simulink model "Skills_Team_15801E_2024"  (R2023a)
settings: Solver=FixedStepAuto  StartTime=0.0  StopTime=inf  RelTol=1e-3
libraries: vexv5lib x45, vexcommonlib x3, slpidlib x2
settings Model: Creator=ctwildnauer24  LastModifiedBy=kevans
settings OptimizationCC: EnhancedBackFolding=on  PassReuseOutputArgsAs=Individual arguments  ZeroExternalMemoryAtStartup=off  ZeroInternalMemoryAtStartup=off  MaxStackSize=64  OptimizeBlockOrder=speed  DifferentSizesBufferReuse=on  OptimizationCustomize=off  EfficientTunableParamExpr=on
settings DebuggingCC: ParameterTunabilityLossMsg=error
settings HardwareCC: ProdBitPerPointer=32  ProdBitPerSizeT=32  ProdBitPerPtrDiffT=32  ProdLargestAtomicInteger=Long  ProdLargestAtomicFloat=Double  ProdWordSize=32  ProdHWDeviceType=ARM Compatible->ARM Cortex  UseEmbeddedCoderFeatures=off
settings SFSimCC: MATLABDynamicMemAlloc=off
settings RTWCC: Description=Embedded Coder  SystemTargetFile=ert.tlc  HardwareBoard=VEX V5 Robot Brain  TLCOptions="-aInlineSetEventsForThisBaseRateFcn=TLC_FALSE -aSuppressMultiTaskScheduler=TLC_FALSE  -aRateBasedStepFcn=0"  TemplateMakefile=ert_default_tmf  Toolchain=GNU Tools for ARM Embedded Processors
settings CodeAppCC: ForceParamTrailComments=on  IgnoreCustomStorageClasses=off  OperatorAnnotations=on  SimulinkDataObjDesc=on  SFDataObjDesc=on  InsertBlockDesc=on
settings ERTTargetCC: SupportNonInlinedSFcns=on  ExtModeTransport=3  ExtModeStaticAlloc=on  ExtModeStaticAllocSize=2048  ExtModeMexFile=ext_xcp  ExtModeIntrfLevel=Level2 - Open

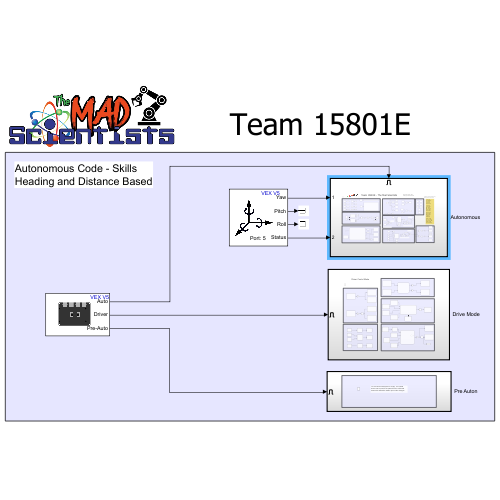
[thumbnail: Simulink's stored preview of the top-level diagram]
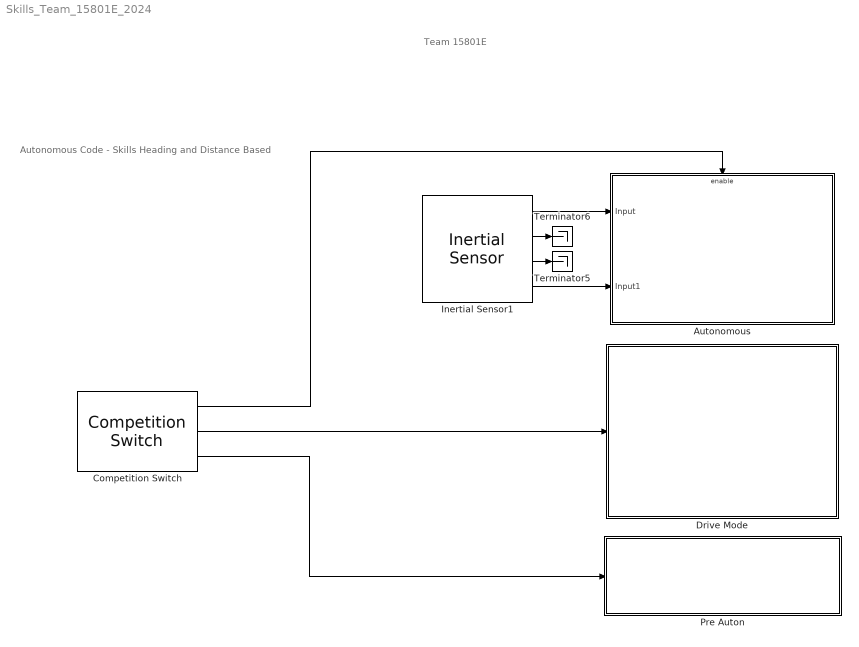
== system Skills_Team_15801E_2024 ==
  note: Team 15801E
  note: Autonomous Code - Skills
      | Heading and Distance Based
  "Autonomous " : Subsystem  TreatAsAtomicUnit=on
  Competition Switch : vexv5lib/Gamepad/Competition Switch  SampleTime=0.02
  "Drive Mode " : Subsystem  TreatAsAtomicUnit=on
  Inertial Sensor1 : vexv5lib/Sensors/Inertial Sensor  Port=5  ypr=on  Quat=off  AngVel=off  Accel=off  CalibStatus=on  YawResetOption=No reset  YawWrapAround=No wrap around  SampleTime=.01
  Pre Auton : Subsystem  TreatAsAtomicUnit=on
  Terminator5 : Terminator
  Terminator6 : Terminator
  wires:
  Competition Switch/2 -> "Drive Mode "/Enable
  Competition Switch/3 -> Pre Auton/Enable
  Competition Switch/1 -> "Autonomous "/Enable
  Inertial Sensor1/3 -> Terminator5/1
  Inertial Sensor1/2 -> Terminator6/1
  Inertial Sensor1/4 -> "Autonomous "/2(Input1)
  Inertial Sensor1/1 -> "Autonomous "/1(Input)

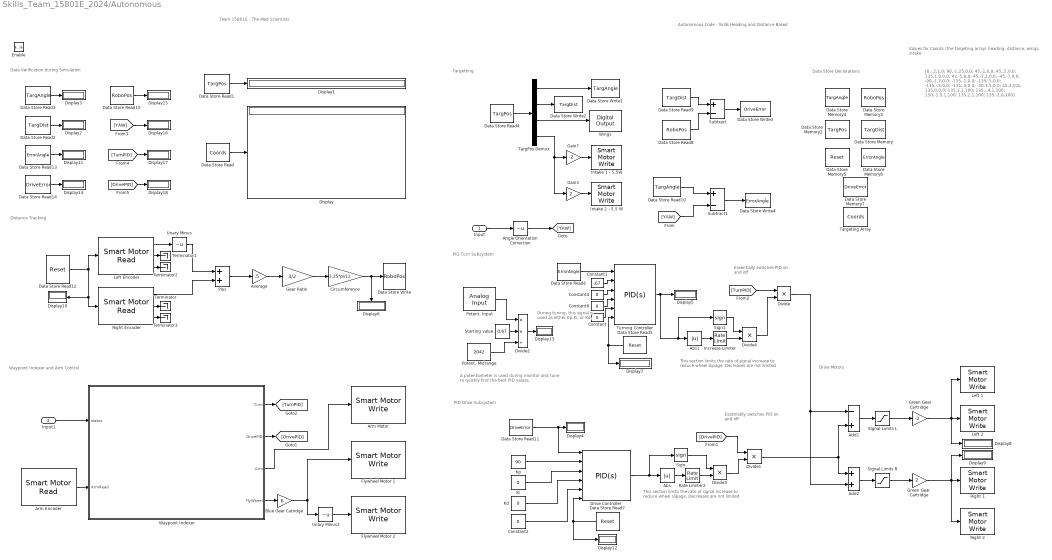
== system Skills_Team_15801E_2024/Autonomous  ==
  note: A potentiometer is used during monitor and tune to quickly find the best PID values.
  note: Data Verification during Simulation
  note: Data Store Declarations
  note: Drive Motors
  note: Waypoint Indexer and Arm Control
  note: Distance Tracking
  note: Team 15801E - The Mad Scientists
  note: PID Turn Subsystem
  note: Autonomous Code - Skills
      | Heading and Distance Based
  note: [0,-.2,1,0;
      | 90,-1.25,0,0;
      | 45,-1,0,0;
      | 45,.5,0,0;
      | 135,1.9,0,0;
      | 42,-5,0,0;
      | 45,-3.2,0,0;
      | -45,-7,0,0;
      | -90,-1.7,0,0;
      | -135,-1,0,0;
      | -135,.5,0,0;
      | -135,-.5,0,0;
      | -135,.5,0,0;
      | -30,3.5,0,0;
      | 45,2,0,0;
      | 135,0,0,0;
      | 135,3,1,100;
      | 135,-.4,1,100;
      | 150,-1.5,1,100;
      | 135,2,1,100;
      | 135,-2,0,100]
  note: Targetting
  note: PID Drive Subsystem
  note: Values for Coords (the targeting array)
      | heading, distance, wings, intake
  note: During tuning, this signal is used as either Kp,Ki, or Kd.
  note: This section limits the rate of signal increase to reduce wheel slipage. Decreases are not limited
  note: Essentially switches PID on and off
  note: This section limits the rate of signal increase to reduce wheel slipage. Decreases are not limited
  note: Essentially switches PID on and off
  Input : Inport
  Input1 : Inport  Port=2
  Enable : EnablePort
  - Green Gear Cartridge : Gain  Gain=-2
  Abs : Abs  SaturateOnIntegerOverflow=off
  Abs1 : Abs  SaturateOnIntegerOverflow=off
  Add1 : Sum  Inputs=-+
  Add2 : Sum
  Angle Orientation Correction : UnaryMinus
  Arm Encoder : vexv5lib/Sensors/Smart Motor Read  motorPort=17  EncoderUnit=Degrees  resetOption=No reset  additionalOutput=off  SampleTime=0.2
  Arm Motor : vexv5lib/Actuators/Smart Motor Write  motorPort=17  scaleFactor=36:1  MotorBrakeMode=Coast  OperationMode=Velocity Control
  Average : Gain  Gain=.5
  Blue Gear Catridge : Gain  Gain=6
  Circumference : Gain  Gain=3.25*pi/12
  Constant{,2,4,6} (4 alike) : Constant  Value=0
  Constant1 : Constant  Value=.67
  Data Store Memory : DataStoreMemory  DataStoreName=TargDist  WriteAfterWriteMsg=warning  ShowAdditionalParam=off  OutDataTypeStr=double
  Data Store Memory2 : DataStoreMemory  DataStoreName=TargPos  WriteAfterWriteMsg=warning  InitialValue=[0,0,0,0]  ShowAdditionalParam=off  OutDataTypeStr=double
  Data Store Memory3 : DataStoreMemory  DataStoreName=RoboPos  WriteAfterWriteMsg=warning  InitialValue=[0]  ShowAdditionalParam=off  OutDataTypeStr=double
  Data Store Memory4 : DataStoreMemory  DataStoreName=TargAngle  WriteAfterWriteMsg=warning  ShowAdditionalParam=off
  Data Store Memory5 : DataStoreMemory  DataStoreName=Reset  WriteAfterWriteMsg=warning  ShowAdditionalParam=off  OutDataTypeStr=double
  Data Store Memory6 : DataStoreMemory  DataStoreName=ErrorAngle  WriteAfterWriteMsg=warning  ShowAdditionalParam=off  OutDataTypeStr=double
  Data Store Memory7 : DataStoreMemory  DataStoreName=DriveError  WriteAfterWriteMsg=warning  ShowAdditionalParam=off  OutDataTypeStr=double
  Data Store Read : DataStoreRead  DataStoreName=Coords  IndexOptions=Index vector (dialog)  Indices=1  OutputSizes=1
  Data Store Read1 : DataStoreRead  DataStoreName=TargPos  IndexOptions=Index vector (dialog)  Indices=1  OutputSizes=1
  Data Store Read10 : DataStoreRead  DataStoreName=TargAngle  IndexOptions=Index vector (dialog)  Indices=1  OutputSizes=1
  Data Store Read11 : DataStoreRead  DataStoreName=DriveError  IndexOptions=Index vector (dialog)  Indices=1  OutputSizes=1
  Data Store Read12 : DataStoreRead  DataStoreName=Reset  IndexOptions=Index vector (dialog)  Indices=1  OutputSizes=1
  Data Store Read13 : DataStoreRead  DataStoreName=ErrorAngle  IndexOptions=Index vector (dialog)  Indices=1  OutputSizes=1
  Data Store Read14 : DataStoreRead  DataStoreName=DriveError  IndexOptions=Index vector (dialog)  Indices=1  OutputSizes=1
  Data Store Read15 : DataStoreRead  DataStoreName=RoboPos  IndexOptions=Index vector (dialog)  Indices=1  OutputSizes=1
  Data Store Read2 : DataStoreRead  DataStoreName=TargDist  IndexOptions=Index vector (dialog)  Indices=1  OutputSizes=1
  Data Store Read3 : DataStoreRead  DataStoreName=TargAngle  IndexOptions=Index vector (dialog)  Indices=1  OutputSizes=1
  Data Store Read4 : DataStoreRead  DataStoreName=TargPos  IndexOptions=Index vector (dialog)  Indices=1  OutputSizes=1
  Data Store Read5 : DataStoreRead  DataStoreName=Reset  IndexOptions=Index vector (dialog)  Indices=1  OutputSizes=1
  Data Store Read6 : DataStoreRead  DataStoreName=ErrorAngle  IndexOptions=Index vector (dialog)  Indices=1  OutputSizes=1
  Data Store Read7 : DataStoreRead  DataStoreName=Reset  IndexOptions=Index vector (dialog)  Indices=1  OutputSizes=1
  Data Store Read8 : DataStoreRead  DataStoreName=RoboPos  IndexOptions=Index vector (dialog)  Indices=1  OutputSizes=1
  Data Store Read9 : DataStoreRead  DataStoreName=TargDist  IndexOptions=Index vector (dialog)  Indices=1  OutputSizes=1
  Data Store Write : DataStoreWrite  DataStoreName=RoboPos  IndexOptions=Index vector (dialog)  Indices=1  OutputSizes=1
  Data Store Write1 : DataStoreWrite  DataStoreName=TargAngle  IndexOptions=Index vector (dialog)  Indices=1  OutputSizes=1
  Data Store Write2 : DataStoreWrite  DataStoreName=TargDist  IndexOptions=Index vector (dialog)  Indices=1  OutputSizes=1
  Data Store Write3 : DataStoreWrite  DataStoreName=DriveError  IndexOptions=Index vector (dialog)  Indices=1  OutputSizes=1
  Data Store Write4 : DataStoreWrite  DataStoreName=ErrorAngle  IndexOptions=Index vector (dialog)  Indices=1  OutputSizes=1
  Display{,1..18} (19 alike) : Display
  Divide{,1,3..4} (4 alike) : Product  Inputs=**
  Divide2 : Product  Inputs=**/
  Drive Controller : slpidlib/PID Controller  Controller=PID  Form=Parallel  TimeDomain=Continuous-time  UseExternalTs=off  SampleTime=-1  IntegratorMethod=Forward Euler  FilterMethod=Forward Euler  ControllerParametersSource=external  P=40  I=0  UseKiTs=off  D=0  N=100  UseFilter=on  TunerSelectOption=Transfer Function Based (PID Tuner App)  InitialConditionSource=internal  InitialConditionForIntegrator=0  InitialConditionForFilter=0  DifferentiatorICPrevScaledInput=0  ExternalReset=either  TrackingMode=off  Kt=1  LimitOutput=on  SatLimitsSource=internal  UpperSaturationLimit=100  LowerSaturationLimit=-100  LinearizeAsGain=on  AntiWindupMode=none  Kb=1  LimitIntegrator=off  UpperIntegratorSaturationLimit=inf  LowerIntegratorSaturationLimit=-inf  POutMin=[]  POutMax=[]  IOutMin=[]  IOutMax=[]  DOutMin=[]  DOutMax=[]  NOutMin=[]  NOutMax=[]  SumOutMin=[]  SumOutMax=[]  SaturationOutMin=[]  SaturationOutMax=[]  PParamMin=[]  PParamMax=[]  IParamMin=[]  IParamMax=[]  DParamMin=[]  DParamMax=[]  NParamMin=[]  NParamMax=[]  KbParamMin=[]  KbParamMax=[]  KtParamMin=[]  KtParamMax=[]  KbOutMin=[]  KbOutMax=[]  KtOutMin=[]  KtOutMax=[]  IntegratorOutMin=[]  IntegratorOutMax=[]  FilterOutMin=[]  FilterOutMax=[]  SumI1OutMin=[]  SumI1OutMax=[]  SumI2OutMin=[]  SumI2OutMax=[]  SumI3OutMin=[]  SumI3OutMax=[]  SumI4OutMin=[]  SumI4OutMax=[]  SumDOutMin=[]  SumDOutMax=[]  DifferentiatorOutMin=[]  DifferentiatorOutMax=[]  FilterDiffOutCoefMin=[]  FilterDiffOutCoefMax=[]  ReciprocalOutMin=[]  ReciprocalOutMax=[]  SumDenOutMin=[]  SumDenOutMax=[]  SumNumOutMin=[]  SumNumOutMax=[]  DivideOutMin=[]  DivideOutMax=[]  UdiffTsProdOutMin=[]  UdiffTsProdOutMax=[]  NTsProdOutMin=[]  NTsProdOutMax=[]  UintegralTsProdOutMin=[]  UintegralTsProdOutMax=[]  UngainTsProdOutMin=[]  UngainTsProdOutMax=[]  ClampingZeroOutDataTypeStr=Inherit: Inherit via back propagation  ClampingZeroOutMin=[]  ClampingZeroOutMax=[]  FilterDenConstantOutDataTypeStr=Inherit: Inherit via back propagation  FilterDenConstantOutMin=[]  FilterDenConstantOutMax=[]  PCopyOutDataTypeStr=Inherit: Inherit via back propagation  PCopyOutMin=[]  PCopyOutMax=[]  NCopyOutDataTypeStr=Inherit: Inherit via back propagation  NCopyOutMin=[]  NCopyOutMax=[]  IntegratorContinuousStateAttributes=''  IntegratorStateMustResolveToSignalObject=off  IntegratorRTWStateStorageClass=Auto  FilterContinuousStateAttributes=''  FilterStateMustResolveToSignalObject=off  FilterRTWStateStorageClass=Auto  ParallelPVariant=ExternalParameters  IdealPVariant=Disabled  IVariant=ExternalParameters  DVariant=ExternalParameters  IntegratorVariant=Continuous  SatVariant=Enabled  AWVariant=Passthrough  PCopyVariant=Disabled  TRVariant=Disabled  FdbkBlocksVariant=Forward  IdealPFdbkVariant=Disabled  SatFdbkVariant=Disabled  DerivativeFilterVariant=ContFilter  NVariant=ExternalParameters  NCopyVariant=Disabled  FilterICVariant=InternalICsFilter  IntegratorICVariant=InternalICs  ExternalResetVariant=ExternalReset  TRSumVariant=Passthrough  SumFdbkVariant=Disabled  SumVariant=Sum_PID  TsampFilterVariant=InternalTs  TsampNgainVariant=Passthrough  TsampIntegralVariant=Disabled_SignalSpec  ExternalSaturationOutDataTypeStr=Inherit: Same as second input
  Flywheel Motor 1 : vexv5lib/Actuators/Smart Motor Write  motorPort=9  scaleFactor=6:1  MotorBrakeMode=Coast  OperationMode=Velocity Control
  Flywheel Motor 2 : vexv5lib/Actuators/Smart Motor Write  motorPort=20  scaleFactor=6:1  MotorBrakeMode=Coast  OperationMode=Velocity Control
  Gain3 : Gain  Gain=2
  Gain7 : Gain  Gain=-2
  Gear Ratio : Gain  Gain=3/2
  Green Gear Cartridge : Gain  Gain=2
  Increase Limiter : RateLimiter  RisingSlewLimit=80  FallingSlewLimit=-1000000  SampleTimeMode=inherited
  Intake 1 - 5.5W : vexv5lib/Actuators/Smart Motor Write  motorPort=11  scaleFactor=18:1  MotorBrakeMode=Coast  OperationMode=Velocity Control
  Intake 2 - 5.5 W : vexv5lib/Actuators/Smart Motor Write  motorPort=3  scaleFactor=18:1  MotorBrakeMode=Coast  OperationMode=Velocity Control
  Kd : Constant  Value=0
  Ki : Constant  Value=0
  Kp : Constant  Value=90
  Left 1 : vexv5lib/Actuators/Smart Motor Write  motorPort=4  scaleFactor=18:1  MotorBrakeMode=Brake  OperationMode=Velocity Control
  Left 2 : vexv5lib/Actuators/Smart Motor Write  motorPort=1  scaleFactor=18:1  MotorBrakeMode=Brake  OperationMode=Velocity Control
  Left Encoder : vexv5lib/Sensors/Smart Motor Read  motorPort=1  EncoderUnit=Rotations  resetOption=Reset by external signal  additionalOutput=on  SampleTime=.01
  Plus : Sum
  Potent. Input : vexv5lib/Sensors/Analog Input  smartPort3wire=None  port=D  SampleTime=0.2
  Potent. Midrange : Constant  Value=2042
  Rate Limiter2 : RateLimiter  RisingSlewLimit=80  FallingSlewLimit=-1000000  SampleTimeMode=inherited
  Right 1 : vexv5lib/Actuators/Smart Motor Write  motorPort=8  scaleFactor=18:1  MotorBrakeMode=Brake  OperationMode=Velocity Control
  Right 2 : vexv5lib/Actuators/Smart Motor Write  motorPort=7  scaleFactor=18:1  MotorBrakeMode=Brake  OperationMode=Velocity Control
  Right Encoder : vexv5lib/Sensors/Smart Motor Read  motorPort=8  EncoderUnit=Rotations  resetOption=Reset by external signal  additionalOutput=on  SampleTime=.01
  Sign : Signum
  Sign1 : Signum
  Signal Limits L : Saturate  UpperLimit=100  LowerLimit=-100
  Signal Limits R : Saturate  UpperLimit=100  LowerLimit=-100
  Starting value : Constant  Value=0.67
  Subtract : Sum  Inputs=+-
  Subtract1 : Sum  Inputs=+-
  TargPos Demux : Demux
  Targeting Array : DataStoreMemory  DataStoreName=Coords  WriteAfterWriteMsg=warning  InitialValue=|  ShowAdditionalParam=off  OutDataTypeStr=double
      | [0,-.2,1,0;
      | 90,-1.25,0,0;
      | 45,-1,0,0;
      | 45,.5,0,0;
      | 135,1.9,0,0;
      | 42,-5,0,0;
      | 45,-3.2,0,0;
      | -45,-7,0,0;
      | -90,-1.7,0,0;
      | -135,-1,0,0;
      | -135,.5,0,0;
      | -135,-.5,0,0;
      | -135,.5,0,0;
      | -30,3.5,0,0;
      | 45,2,0,0;
      | 135,0,0,0;
      | 135,3,1,100;
      | 135,-.4,1,100;
      | 150,-1.5,1,100;
      | 135,2,1,100;
      | 135,-2,0,100]
  Terminator{,1..3} (4 alike) : Terminator
  Turning Controller : slpidlib/PID Controller  Controller=PID  Form=Parallel  TimeDomain=Continuous-time  UseExternalTs=off  SampleTime=-1  IntegratorMethod=Forward Euler  FilterMethod=Forward Euler  ControllerParametersSource=external  P=.4  I=0  UseKiTs=off  D=0  N=100  UseFilter=on  TunerSelectOption=Transfer Function Based (PID Tuner App)  InitialConditionSource=internal  InitialConditionForIntegrator=0  InitialConditionForFilter=0  DifferentiatorICPrevScaledInput=0  ExternalReset=either  TrackingMode=off  Kt=1  LimitOutput=on  SatLimitsSource=internal  UpperSaturationLimit=100  LowerSaturationLimit=-100  LinearizeAsGain=on  AntiWindupMode=none  Kb=1  LimitIntegrator=off  UpperIntegratorSaturationLimit=inf  LowerIntegratorSaturationLimit=-inf  POutMin=[]  POutMax=[]  IOutMin=[]  IOutMax=[]  DOutMin=[]  DOutMax=[]  NOutMin=[]  NOutMax=[]  SumOutMin=[]  SumOutMax=[]  SaturationOutMin=[]  SaturationOutMax=[]  PParamMin=[]  PParamMax=[]  IParamMin=[]  IParamMax=[]  DParamMin=[]  DParamMax=[]  NParamMin=[]  NParamMax=[]  KbParamMin=[]  KbParamMax=[]  KtParamMin=[]  KtParamMax=[]  KbOutMin=[]  KbOutMax=[]  KtOutMin=[]  KtOutMax=[]  IntegratorOutMin=[]  IntegratorOutMax=[]  FilterOutMin=[]  FilterOutMax=[]  SumI1OutMin=[]  SumI1OutMax=[]  SumI2OutMin=[]  SumI2OutMax=[]  SumI3OutMin=[]  SumI3OutMax=[]  SumI4OutMin=[]  SumI4OutMax=[]  SumDOutMin=[]  SumDOutMax=[]  DifferentiatorOutMin=[]  DifferentiatorOutMax=[]  FilterDiffOutCoefMin=[]  FilterDiffOutCoefMax=[]  ReciprocalOutMin=[]  ReciprocalOutMax=[]  SumDenOutMin=[]  SumDenOutMax=[]  SumNumOutMin=[]  SumNumOutMax=[]  DivideOutMin=[]  DivideOutMax=[]  UdiffTsProdOutMin=[]  UdiffTsProdOutMax=[]  NTsProdOutMin=[]  NTsProdOutMax=[]  UintegralTsProdOutMin=[]  UintegralTsProdOutMax=[]  UngainTsProdOutMin=[]  UngainTsProdOutMax=[]  ClampingZeroOutDataTypeStr=Inherit: Inherit via back propagation  ClampingZeroOutMin=[]  ClampingZeroOutMax=[]  FilterDenConstantOutDataTypeStr=Inherit: Inherit via back propagation  FilterDenConstantOutMin=[]  FilterDenConstantOutMax=[]  PCopyOutDataTypeStr=Inherit: Inherit via back propagation  PCopyOutMin=[]  PCopyOutMax=[]  NCopyOutDataTypeStr=Inherit: Inherit via back propagation  NCopyOutMin=[]  NCopyOutMax=[]  IntegratorContinuousStateAttributes=''  IntegratorStateMustResolveToSignalObject=off  IntegratorRTWStateStorageClass=Auto  FilterContinuousStateAttributes=''  FilterStateMustResolveToSignalObject=off  FilterRTWStateStorageClass=Auto  ParallelPVariant=ExternalParameters  IdealPVariant=Disabled  IVariant=ExternalParameters  DVariant=ExternalParameters  IntegratorVariant=Continuous  SatVariant=Enabled  AWVariant=Passthrough  PCopyVariant=Disabled  TRVariant=Disabled  FdbkBlocksVariant=Forward  IdealPFdbkVariant=Disabled  SatFdbkVariant=Disabled  DerivativeFilterVariant=ContFilter  NVariant=ExternalParameters  NCopyVariant=Disabled  FilterICVariant=InternalICsFilter  IntegratorICVariant=InternalICs  ExternalResetVariant=ExternalReset  TRSumVariant=Passthrough  SumFdbkVariant=Disabled  SumVariant=Sum_PID  TsampFilterVariant=InternalTs  TsampNgainVariant=Passthrough  TsampIntegralVariant=Disabled_SignalSpec  ExternalSaturationOutDataTypeStr=Inherit: Same as second input
  Unary Minus : UnaryMinus
  Unary Minus3 : UnaryMinus
  Waypoint Indexer : Stateflow chart  TreatAsAtomicUnit=on
  Wings : vexv5lib/Actuators/Digital Output  smartPort3wire=None  port=B
  wires:
  Subtract/1 -> Data Store Write3/1
  Waypoint Indexer/3(Arm) -> Arm Motor/1
  - Green Gear Cartridge/1 -> Left 1/1, Left 2/1, Display8/1
  Arm Encoder/1 -> Waypoint Indexer/2(ArmRead)
  Data Store Read1/1 -> Display1/1
  Sign/1 -> Divide3/1
  Data Store Read6/1 -> Turning Controller/1
  Divide/1 -> Add2/2, Add1/1
  [TurnPID] -> Divide/1
  Increase Limiter/1 -> Divide4/2
  Add1/1 -> Signal Limits L/1
  Right Encoder/2 -> Terminator/1
  Data Store Read3/1 -> Display3/1
  Divide4/1 -> Divide/2
  Constant1/1 -> Turning Controller/2
  Starting value/1 -> Divide2/2
  TargPos Demux/2 -> Data Store Write2/1
  Divide2/1 -> Display13/1
  Circumference/1 -> Data Store Write/1, Display6/1
  Data Store Read11/1 -> Display4/1, Drive Controller/1
  Kd/1 -> Drive Controller/4
  Data Store Read/1 -> Display/1
  Abs/1 -> Rate Limiter2/1
  Constant4/1 -> Turning Controller/3
  Waypoint Indexer/1(Turn) -> [TurnPID]
  Potent. Midrange/1 -> Divide2/3
  Ki/1 -> Drive Controller/3
  Divide1/1 -> Add2/1, Add1/2
  Turning Controller/1 -> Sign1/1, Abs1/1, Display5/1
  Data Store Read2/1 -> Display2/1
  [DrivePID] -> Divide1/1
  Potent. Input/1 -> Divide2/1
  Data Store Read10/1 -> Subtract1/1
  Kp/1 -> Drive Controller/2
  Left Encoder/2 -> Terminator1/1
  Subtract1/1 -> Data Store Write4/1
  Rate Limiter2/1 -> Divide3/2
  Data Store Read5/1 -> Turning Controller/6, Display7/1
  TargPos Demux/1 -> Data Store Write1/1
  Plus/1 -> Average/1
  Data Store Read9/1 -> Subtract/1
  Waypoint Indexer/2(DrivePID) -> [DrivePID]
  Abs1/1 -> Increase Limiter/1
  Average/1 -> Gear Ratio/1
  Data Store Read8/1 -> Subtract/2
  Gear Ratio/1 -> Circumference/1
  Signal Limits R/1 -> Green Gear Cartridge/1
  Data Store Read12/1 -> Right Encoder/1, Display10/1, Left Encoder/1
  Add2/1 -> Signal Limits R/1
  Unary Minus/1 -> Plus/1
  Green Gear Cartridge/1 -> Display9/1, Right 1/1, Right 2/1
  Angle Orientation Correction/1 -> [YAW]
  Left Encoder/1 -> Unary Minus/1
  Left Encoder/3 -> Terminator2/1
  Right Encoder/3 -> Terminator3/1
  Drive Controller/1 -> Sign/1, Abs/1
  TargPos Demux/4 -> Gain3/1, Gain7/1
  TargPos Demux/3 -> Wings/1
  Signal Limits L/1 -> - Green Gear Cartridge/1
  Data Store Read4/1 -> TargPos Demux/1
  Divide3/1 -> Divide1/2
  Constant6/1 -> Turning Controller/4
  Data Store Read7/1 -> Drive Controller/6, Display12/1
  Gain3/1 -> Intake 2 - 5.5 W/1
  Gain7/1 -> Intake 1 - 5.5W/1
  [YAW] -> Subtract1/2
  Sign1/1 -> Divide4/1
  Right Encoder/1 -> Plus/2
  Input/1 -> Angle Orientation Correction/1
  Input1/1 -> Waypoint Indexer/1(status)
  Constant/1 -> Turning Controller/5
  Constant2/1 -> Drive Controller/5
  Waypoint Indexer/4(FlyWheel) -> Blue Gear Catridge/1
  Blue Gear Catridge/1 -> Unary Minus3/1, Flywheel Motor 1/1
  Unary Minus3/1 -> Flywheel Motor 2/1
  Data Store Read14/1 -> Display14/1
  Data Store Read13/1 -> Display11/1
  Data Store Read15/1 -> Display15/1
  [YAW] -> Display16/1
  [TurnPID] -> Display17/1
  [DrivePID] -> Display18/1

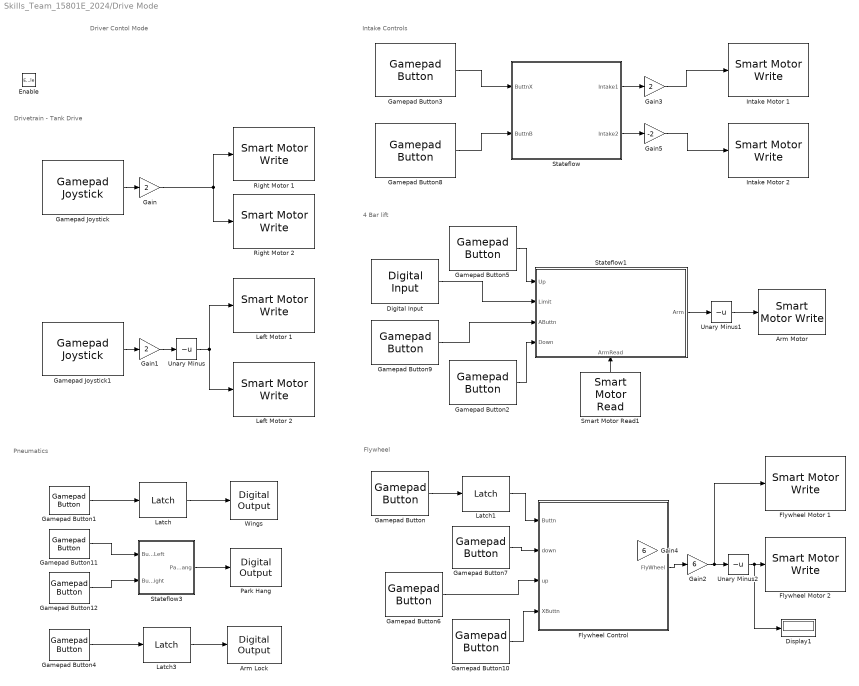
== system Skills_Team_15801E_2024/Drive Mode  ==
  note: Driver Contol Mode
  note: Flywheel
  note: 4 Bar lift
  note: Pneumatics
  note: Intake Controls
  note: Drivetrain - Tank Drive
  Enable : EnablePort
  Arm Lock : vexv5lib/Actuators/Digital Output  smartPort3wire=None  port=E
  Arm Motor : vexv5lib/Actuators/Smart Motor Write  motorPort=17  scaleFactor=36:1  MotorBrakeMode=Brake  OperationMode=Velocity Control
  Digital Input : vexv5lib/Sensors/Digital Input  smartPort3wire=None  port=C  SampleTime=0.2
  Display1 : Display
  Flywheel Control : Stateflow chart  TreatAsAtomicUnit=on
  Flywheel Motor 1 : vexv5lib/Actuators/Smart Motor Write  motorPort=9  scaleFactor=6:1  MotorBrakeMode=Coast  OperationMode=Velocity Control
  Flywheel Motor 2 : vexv5lib/Actuators/Smart Motor Write  motorPort=20  scaleFactor=6:1  MotorBrakeMode=Coast  OperationMode=Velocity Control
  Gain : Gain  Gain=2
  Gain1 : Gain  Gain=2
  Gain2 : Gain  Gain=6
  Gain3 : Gain  Gain=2
  Gain4 : Gain  Gain=6
  Gain5 : Gain  Gain=-2
  Gamepad Button : vexv5lib/Gamepad/Gamepad Button  joystickType=Primary  chan=A  SampleTime=0.02
  Gamepad Button1 : vexv5lib/Gamepad/Gamepad Button  joystickType=Primary  chan=Y  SampleTime=0.02
  Gamepad Button10 : vexv5lib/Gamepad/Gamepad Button  joystickType=Primary  chan=X  SampleTime=0.02
  Gamepad Button11 : vexv5lib/Gamepad/Gamepad Button  joystickType=Primary  chan=LEFT  SampleTime=0.02
  Gamepad Button12 : vexv5lib/Gamepad/Gamepad Button  joystickType=Primary  chan=RIGHT  SampleTime=0.02
  Gamepad Button2 : vexv5lib/Gamepad/Gamepad Button  joystickType=Primary  chan=L1  SampleTime=0.02
  Gamepad Button3 : vexv5lib/Gamepad/Gamepad Button  joystickType=Primary  chan=R2  SampleTime=0.02
  Gamepad Button4 : vexv5lib/Gamepad/Gamepad Button  joystickType=Primary  chan=B  SampleTime=0.02
  Gamepad Button5 : vexv5lib/Gamepad/Gamepad Button  joystickType=Primary  chan=L2  SampleTime=0.02
  Gamepad Button6 : vexv5lib/Gamepad/Gamepad Button  joystickType=Primary  chan=UP  SampleTime=0.02
  Gamepad Button7 : vexv5lib/Gamepad/Gamepad Button  joystickType=Primary  chan=DOWN  SampleTime=0.02
  Gamepad Button8 : vexv5lib/Gamepad/Gamepad Button  joystickType=Primary  chan=R1  SampleTime=0.02
  Gamepad Button9 : vexv5lib/Gamepad/Gamepad Button  joystickType=Primary  chan=B  SampleTime=0.02
  Gamepad Joystick : vexv5lib/Gamepad/Gamepad Joystick  joystickType=Primary  chan=2  SampleTime=0.02
  Gamepad Joystick1 : vexv5lib/Gamepad/Gamepad Joystick  joystickType=Primary  chan=3  SampleTime=0.02
  Intake Motor 1 : vexv5lib/Actuators/Smart Motor Write  motorPort=3  scaleFactor=18:1  MotorBrakeMode=Coast  OperationMode=Velocity Control
  Intake Motor 2 : vexv5lib/Actuators/Smart Motor Write  motorPort=11  scaleFactor=18:1  MotorBrakeMode=Coast  OperationMode=Velocity Control
  Latch : vexcommonlib/Latch  output0=off  BlockPlatform=vexarmcortex
      settings: LibrarySourceBlock=vexarmcortexlib/Utilities/Latch
  Latch1 : vexcommonlib/Latch  output0=off  BlockPlatform=vexarmcortex
      settings: LibrarySourceBlock=vexarmcortexlib/Utilities/Latch
  Latch3 : vexcommonlib/Latch  output0=off  BlockPlatform=vexarmcortex
      settings: LibrarySourceBlock=vexarmcortexlib/Utilities/Latch
  Left Motor 1 : vexv5lib/Actuators/Smart Motor Write  motorPort=4  scaleFactor=18:1  MotorBrakeMode=Brake  OperationMode=Velocity Control
  Left Motor 2 : vexv5lib/Actuators/Smart Motor Write  motorPort=1  scaleFactor=18:1  MotorBrakeMode=Brake  OperationMode=Velocity Control
  Park Hang : vexv5lib/Actuators/Digital Output  smartPort3wire=None  port=H
  Right Motor 1 : vexv5lib/Actuators/Smart Motor Write  motorPort=8  scaleFactor=18:1  MotorBrakeMode=Brake  OperationMode=Velocity Control
  Right Motor 2 : vexv5lib/Actuators/Smart Motor Write  motorPort=7  scaleFactor=18:1  MotorBrakeMode=Brake  OperationMode=Velocity Control
  Smart Motor Read1 : vexv5lib/Sensors/Smart Motor Read  motorPort=17  EncoderUnit=Degrees  resetOption=No reset  additionalOutput=off  SampleTime=0.2
  Stateflow : Stateflow chart  TreatAsAtomicUnit=on
  Stateflow1 : Stateflow chart  TreatAsAtomicUnit=on
      settings: PortSchema="{\"entries\":[{\"content\":{\"sides\":[{\"content\":{\"connectorIds\":[\"In2\",\"In3\",\"In4\",\"In1\"]},\"type\":\"ConnectorPlacement.EquallySpacedRectSide\",\"uuid\":\"b847d8da-5a24-44a0-8083-9d48600015b9\"},{\"content\":{\"connectorIds\":[\"Out1\"],\"side\":\"RIGHT\"},\"type\":\"ConnectorPlacement.EquallySpacedRectSide\",\"uuid\":\"9ccdf8c1-91e9-479a-b3b5-791405739968\"},{\"content\":{\"side\":\"TOP\"},\"type\":\"ConnectorPlacement.EquallySpacedRectSide\",\"uuid\":\"e64e2570-37d5-4b4f-b532-f4d53c4496c9\"},{\"content\":{\"connectorIds\":[\"In5\"],\"side\":\"BOTTOM\"},\"type\":\"ConnectorPlacement.EquallySpacedRectSide\",\"uuid\":\"786147ef-6ec2-46ae-a68d-f295a13af8d8\"}]},\"type\":\"ConnectorPlacement.EquallySpacedConnector\",\"uuid\":\"6648d0de-94c0-4657-b42d-3f591035da08\"}],\"packageUris\":[\"http://schema.mathworks.com/mf0/Connector/R2020b\"],\"version\":\"1.0\"}"
  Stateflow3 : Stateflow chart  TreatAsAtomicUnit=on
  Unary Minus : UnaryMinus
  Unary Minus1 : UnaryMinus
  Unary Minus2 : UnaryMinus
  Wings : vexv5lib/Actuators/Digital Output  smartPort3wire=None  port=B
  wires:
  Gain/1 -> Right Motor 1/1, Right Motor 2/1
  Stateflow1/1(Arm) -> Unary Minus1/1
  Unary Minus/1 -> Left Motor 2/1, Left Motor 1/1
  Stateflow3/1(ParkHang) -> Park Hang/1
  Gamepad Button3/1 -> Stateflow/1(ButtnX)
  Gamepad Button12/1 -> Stateflow3/2(ButtnRight)
  Gamepad Button11/1 -> Stateflow3/1(ButtnLeft)
  Gamepad Button10/1 -> Flywheel Control/4(XButtn)
  Gamepad Button9/1 -> Stateflow1/4(AButtn)
  Stateflow/2(Intake2) -> Gain5/1
  Gamepad Button1/1 -> Latch/1
  Latch/1 -> Wings/1
  Latch1/1 -> Flywheel Control/1(Buttn)
  Gamepad Button4/1 -> Latch3/1
  Gamepad Button5/1 -> Stateflow1/2(Up)
  Smart Motor Read1/1 -> Stateflow1/5(ArmRead)
  Stateflow/1(Intake1) -> Gain3/1
  Gamepad Button7/1 -> Flywheel Control/2(down)
  Gamepad Button8/1 -> Stateflow/2(ButtnB)
  Unary Minus1/1 -> Arm Motor/1
  Unary Minus2/1 -> Display1/1, Flywheel Motor 2/1
  Gamepad Button/1 -> Latch1/1
  Gain3/1 -> Intake Motor 1/1
  Gain1/1 -> Unary Minus/1
  Gamepad Joystick/1 -> Gain/1
  Gamepad Button6/1 -> Flywheel Control/3(up)
  Gamepad Button2/1 -> Stateflow1/1(Down)
  Flywheel Control/1(FlyWheel) -> Gain2/1
  Gain5/1 -> Intake Motor 2/1
  Gain2/1 -> Flywheel Motor 1/1, Unary Minus2/1
  Digital Input/1 -> Stateflow1/3(Limit)
  Latch3/1 -> Arm Lock/1
  Gamepad Joystick1/1 -> Gain1/1

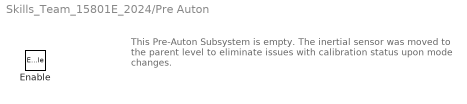
== system Skills_Team_15801E_2024/Pre Auton ==
  note: This Pre-Auton Subsystem is empty. The inertial sensor was moved to the parent level to eliminate issues with calibration status upon mode changes.
  Enable : EnablePort

== stateflow chart Skills_Team_15801E_2024/Drive Mode /Stateflow ==
  state Off
    Intake1=0;
    Intake2=0;
  state Out
    Intake1=-100;
    Intake2=-100;
  state In
    Intake1=100;
    Intake2=100;
  (default) -> Off
  Off -> Out [order 2] : [ButtnX==0 && ButtnB==1]
  Off -> In [order 1] : [ButtnX==1 && ButtnB==0]
  Out -> Off : [ButtnX==0 && ButtnB==0 || ButtnX==1 && ButtnB==1]
  In -> Off : [ButtnX==0 && ButtnB==0 || ButtnX==1 && ButtnB==1]
  data: ButtnX input; Intake1 output; Intake2 output; ButtnB input

== stateflow chart Skills_Team_15801E_2024/Autonomous /Waypoint Indexer ==
  note: The first staeflow chart controls how the robot progresses through each portion of the autonomous routine. Once each target has been reached, PID and encoder counts are reset before the target is updated to the next element of the targetting array.
  note: The second staeflow chart raises the arm into launch position and them lowers back down so th erobot can go under the elvation bar.
  state Coordinates [parallel]
    settings: executionOrder=1
    state start
      dim=size(Coords);
      max=dim(1);
      FlyWheel=0;
    note: The size of the target array is determined so the code halts at the final target.
    state Calibrate
    note: The current target is stored at TargPos
    state Targeting
      TargPos = transpose(Coords(index,:));
    state Reset1
      Reset=1;
    note: Turning PID - ON; Driving PID - OFF
    state Shoot
      FlyWheel=100;
    state turnOn
      Reset=0;
      Turn=1;
      DrivePID=0;
    note: Heading Reached
    state Reset2
      Reset=1;
    note: Turning PID - OFF; Driving PID - ON
    note: Once the inertial sensor is calinrated, the flywheel is activated for 27.89 seconds.
    state Drive
      entry:
      Reset=0;
      Turn=0;
      DrivePID=1;
    note: Distance Reached
    state Increase_Index
      entry:
      DrivePID=0;
      index=index+1;
    note: Increase Target Index
    Shoot -> start : [after(27.89,sec)]
    (default) -> Calibrate
    start -> Targeting
    Calibrate -> Shoot : [status==1]
    Increase_Index -> Targeting : [index<=max]
    Targeting -> Reset1
    Reset1 -> turnOn
    turnOn -> Reset2 : [abs(ErrorAngle)<=3]
    Reset2 -> Drive
    Drive -> Increase_Index : [abs(DriveError)<=0.05 || after(2,sec)]
  state ArmControl [parallel]
    settings: executionOrder=2
    state Start
      Arm=0;
    state Raise
      Arm=100;
    state Stop
      Arm=0;
    state Lower
      Arm=-100;
    state Stop1
      Arm=0;
    (default) -> Start
    Start -> Raise
    Raise -> Stop : [ArmRead>=370]
    Stop -> Lower : [after(27.89,sec)]
    Lower -> Stop1 : [ArmRead<=10]
  note: The parallel stateflow charts allow for arm control independent of the indexing loop
  (default) -> Coordinates [order 1]
  (default) -> ArmControl [order 2]
  data: dim local; index local double =1; Reset data_store_memory; Coords data_store_memory; max local; TargPos data_store_memory; status input; Turn output; DrivePID output; ErrorAngle data_store_memory; DriveError data_store_memory; Arm output; ArmRead input; FlyWheel output

== stateflow chart Skills_Team_15801E_2024/Drive Mode /Flywheel Control ==
  state OnOff [parallel]
    settings: executionOrder=1
    note: This chart turns the flywheel on and off for launching triballs.
    state Start
      entry:
      FlyWheel=0;
    state On
      FlyWheel=80*(1-.1*gear)
    (default) -> OnOff.Start
    OnOff.Start -> On : [Buttn==1]
    On -> OnOff.Start : [Buttn==0]
  state SpeedTransmission [parallel]
    settings: executionOrder=2
    note: This chart serves as a speed transmission to increase/decrease the flywheel speed. This permits better in-match control of triball placement.
    state down_pressed
    state base
    state up_pressed
    (default) -> base : {gear =0;}
    base -> down_pressed [order 2] : [down~=0 && gear<4]{gear=gear+1;}
    base -> up_pressed [order 1] : [up~=0 && gear>0]{gear=gear-1;}
    down_pressed -> base : [down==0 && gear<=4]
    up_pressed -> base : [up==0 && gear>=0]
  state SpinBackwards [parallel]
    settings: executionOrder=3
    note: This chart runs the flywheel slowly in reverse to aid in matchloading triballs into the intake from the top.
    state Start
      entry:
      FlyWheel=0;
    state Back
      entry:
      FlyWheel=-30;
    (default) -> SpinBackwards.Start
    SpinBackwards.Start -> Back : [XButtn==1 && after(.5,sec)]
    Back -> SpinBackwards.Start : [XButtn==1 && after(.5,sec)]
  data: Buttn input; down input; up input; FlyWheel output; gear local; XButtn input

== stateflow chart Skills_Team_15801E_2024/Drive Mode /Stateflow1 ==
  note: Manual Lift Control - 3 states - Off, Up, & Down
  state Controls [parallel]
    settings: executionOrder=1
    state Off
      entry:
      Arm1=0;
    state Up1
      entry:
      Arm1=-100;
    state Down
      entry:
      Arm1=100;
    (default) -> Off
    Up1 -> Off [order 2] : [Up==0 && Down ==0]
    Controls.Down -> Off [order 2] : [Limit==1|| Up==0 && Down ==0 ]
    Off -> Up1 [order 2] : [Down==1 && Up==0]
    Off -> Controls.Down [order 1] : [Limit==0 && Down==0 && Up==1 ]
    Controls.Down -> Up1 [order 1] : [Down==1 && Up==0]
    Up1 -> Controls.Down [order 1] : [Up==1 && Down==0 && Limit==0]
  state Stop [parallel]
    settings: executionOrder=2
    note: Arm moves either up or down to a predetermined height to matchload by launching of feeding into intake from top. Position still allows for passage under the elevation bar.
    state Stop
      entry:
      Arm2=0;
    state Down
      entry:
      Arm2=100;
    state Up
      entry:
      Arm2=-100;
    (default) -> Stop.Stop
    Stop.Stop -> Up [order 2] : [ArmRead<200 && AButtn==1]
    Stop.Stop -> Stop.Down [order 1] : [ArmRead>=200 && AButtn==1]
    Up -> Stop.Stop : [ArmRead>=370]
    Stop.Down -> Stop.Stop : [ArmRead<=0]
  state ANTIMASH [parallel]
    Arm=Arm1+Arm2;
    settings: executionOrder=3
  note: This third parallel state combines the lift outputs from both systems to prevent issues with manual input while the automaic system is operating.
  data: Down input; Up input; Limit input; AButtn input; ArmRead input; Arm1 local; Arm2 local; Arm output

== stateflow chart Skills_Team_15801E_2024/Drive Mode /Stateflow3 ==
  state Start
    ParkHang=0;
  state Hold
    ParkHang=1;
  (default) -> Start
  Hold -> Start : [ButtnLeft==1 && ButtnRight==0]
  Start -> Hold : [ButtnRight==1 &&  ButtnLeft==0]
  data: ButtnLeft input; ButtnRight input; ParkHang output
